simulink model "TorquecontrolModel"  (R2022a)
settings: Solver=VariableStepAuto  StartTime=0.0  StopTime=10.0  RelTol=1e-3
undefined symbols (not defined in the file): a, b, c, D, J, kii, kpi, kpo, Kt, R, Tc
settings Model: Creator=sokse  LastModifiedBy=sokse

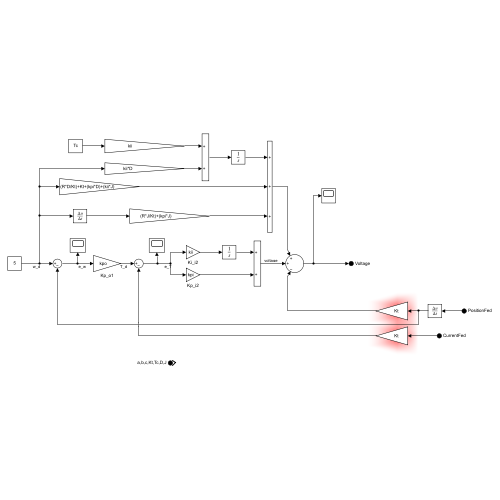
[thumbnail: Simulink's stored preview of the top-level diagram]
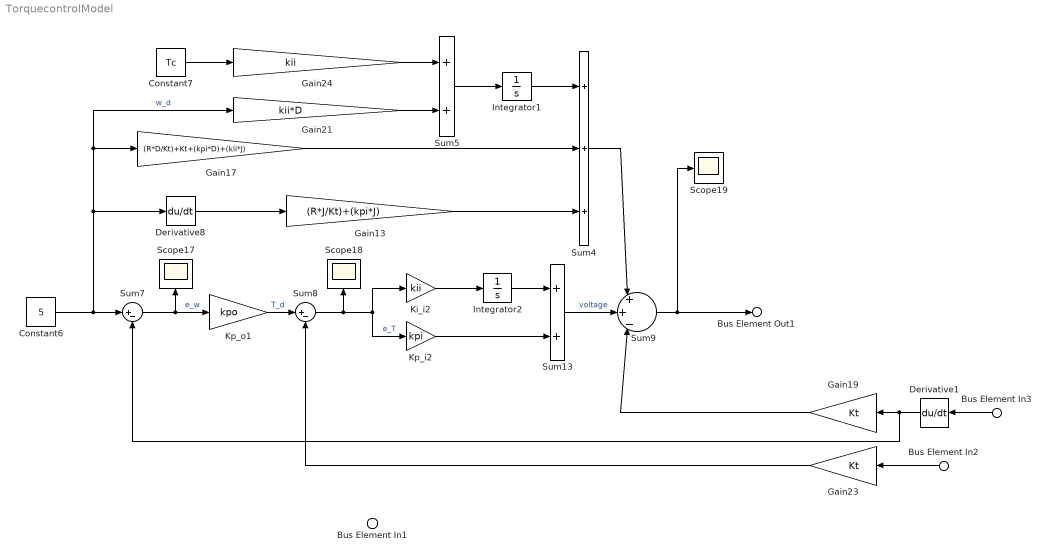
== system TorquecontrolModel ==
  Bus Element In2 : Inport  PortName=CurrentFed
  Bus Element In1 : Inport  Port=2  PortName=a,b,c,Kt,Tc,D,J
  Bus Element In3 : Inport  Port=3  PortName=PositionFed
  Constant6 : Constant  Value=5
  Constant7 : Constant  Value=Tc
  Derivative1 : Derivative
  Derivative8 : Derivative
  Gain13 : Gain  Gain=(R*J/Kt)+(kpi*J)
  Gain17 : Gain  Gain=(R*D/Kt)+Kt+(kpi*D)+(kii*J)
  Gain19 : Gain  Gain=Kt
  Gain21 : Gain  Gain=kii*D
  Gain23 : Gain  Gain=Kt
  Gain24 : Gain  Gain=kii
  Integrator1 : Integrator
  Integrator2 : Integrator
  Ki_i2 : Gain  Gain=kii
  Kp_i2 : Gain  Gain=kpi
  Kp_o1 : Gain  Gain=kpo
  Scope17 : Scope
  Scope18 : Scope
  Scope19 : Scope
  Sum13 : Sum
  Sum4 : Sum  Inputs=+++
  Sum5 : Sum
  Sum7 : Sum  Inputs=|+-
  Sum8 : Sum  Inputs=|+-
  Sum9 : Sum  Inputs=|+|+|-|
  Bus Element Out1 : Outport  PortName=Voltage
  wires:
  Kp_i2/1 -> Sum13/2
  Ki_i2/1 -> Integrator2/1
  Gain13/1 -> Sum4/3
  Kp_o1/1 -> Sum8/1  "T_d"
  Integrator1/1 -> Sum4/1
  Sum7/1 -> Kp_o1/1, Scope17/1  "e_w"
  Gain17/1 -> Sum4/2
  Sum8/1 -> Scope18/1, Kp_i2/1, Ki_i2/1  "e_T"
  Constant7/1 -> Gain24/1
  Sum9/1 -> Bus Element Out1/1, Scope19/1
  Derivative8/1 -> Gain13/1
  Sum5/1 -> Integrator1/1
  Gain21/1 -> Sum5/2
  Sum4/1 -> Sum9/1
  Constant6/1 -> Sum7/1, Derivative8/1, Gain17/1, Gain21/1  "w_d"
  Gain24/1 -> Sum5/1
  Gain23/1 -> Sum8/2
  Integrator2/1 -> Sum13/1
  Sum13/1 -> Sum9/2  "voltage"
  Gain19/1 -> Sum9/3
  Bus Element In3/1 -> Derivative1/1
  Derivative1/1 -> Sum7/2, Gain19/1
  Bus Element In2/1 -> Gain23/1
